simulink model "CASO_EJERCICIO"  (R2019b)
settings: Solver=VariableStepAuto  StartTime=0.0  StopTime=60000  RelTol=1e-3
undefined symbols (not defined in the file): n, p1, p2, p3, Vi
libraries: simulink x12
settings Model: Creator=USUARIO  LastModifiedBy=USUARIO

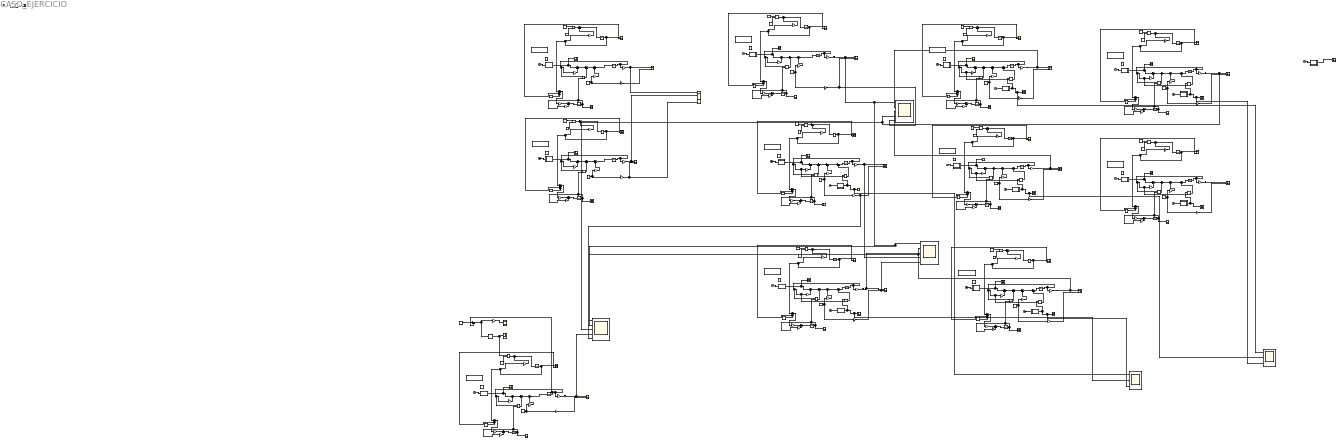
== system CASO_EJERCICIO ==
  COMPARACION MAXIMOS EJERCICIOS PRE Y POST INGESTA : Scope  NumInputPorts=5
  Clock{,1..18,26} (20 alike) : Clock
  Constant{1,3,5,7,9,11,13,15,19,21,29} (11 alike) : Constant  Value=0
  Constant{2,4,6,8,10,12,14,16,20,22,30} (11 alike) : Constant  Value=Vi
  Divide{1..8,10..11,15} (11 alike) : Product  Inputs=*/
  EJERCICIO PREVIO : Scope  NumInputPorts=3
  EJERCICIO TRAS : Scope  NumInputPorts=3
  Error glucémico10 : Scope
  Gain{1,6,8,13,18,20,25,27,32,34,39,41,46,48,53,55,64,68,73,76,105,110} (22 alike) : Gain  Gain=p1
  Gain{3,5,10,12,15,17,22,24,29,31,36,38,43,45,50,52,66,70,72,75,107,109,112} (23 alike) : Gain  Gain=18
  Gain{2,9,21,28,35,42,49,56,65,69,106} (11 alike) : Gain  Gain=p3
  Gain{4,11,16,23,30,37,44,51,67,71,108} (11 alike) : Gain  Gain=n
  Gain{7,14,19,26,33,40,47,54,74,77,111} (11 alike) : Gain  Gain=p2
  Glucosa basal{1..8,10..11,15} (11 alike) : Constant  Value=7
  Grafica ingesta D{1..18,20} (19 alike) : Scope
  Ingesta 75 g1 : MATLAB Function  TreatAsAtomicUnit=on
  Ingesta 75 g10 : MATLAB Function  TreatAsAtomicUnit=on
  Ingesta 75 g11 : MATLAB Function  TreatAsAtomicUnit=on
  Ingesta 75 g15 : MATLAB Function  TreatAsAtomicUnit=on
  Ingesta 75 g2 : MATLAB Function  TreatAsAtomicUnit=on
  Ingesta 75 g3 : MATLAB Function  TreatAsAtomicUnit=on
  Ingesta 75 g4 : MATLAB Function  TreatAsAtomicUnit=on
  Ingesta 75 g5 : MATLAB Function  TreatAsAtomicUnit=on
  Ingesta 75 g6 : MATLAB Function  TreatAsAtomicUnit=on
  Ingesta 75 g7 : MATLAB Function  TreatAsAtomicUnit=on
  Ingesta 75 g8 : MATLAB Function  TreatAsAtomicUnit=on
  Ingesta 75 g9 : MATLAB Function  TreatAsAtomicUnit=on
  Insulina basal{1..8,10..11,15} (11 alike) : Constant  Value=10
  Integrator{1,4,7,10,13,19,22,28,31,43} (10 alike) : Integrator  InitialCondition=10
  Integrator{2,5,8,11,14,17,20,23,29,32,44} (11 alike) : Integrator  InitialCondition=7
  Integrator{3,6,9,12,15..16,18,21,24,30,45} (11 alike) : Integrator
  Integrator33 : Integrator  InitialCondition=-0.000194
  MATLAB Function : MATLAB Function  TreatAsAtomicUnit=on
  MATLAB Function1 : MATLAB Function  TreatAsAtomicUnit=on
  MATLAB Function2 : MATLAB Function  TreatAsAtomicUnit=on
  MATLAB Function3 : MATLAB Function  TreatAsAtomicUnit=on
  MATLAB Function4 : MATLAB Function  TreatAsAtomicUnit=on
  MATLAB Function5 : MATLAB Function  TreatAsAtomicUnit=on
  MATLAB Function6 : MATLAB Function  TreatAsAtomicUnit=on
  MATLAB Function7 : MATLAB Function  TreatAsAtomicUnit=on
  Model Info1 : simulink/Model-Wide Utilities/Model Info  Frame=on  DisplayStringWithTags=|  HorizontalTextAlignment=Center  LeftAlignmentValue=0.5
      | MODELO MODIFICADO
      | 
      | INGESTA SIN INSULINA
      | 
      | PERSONA DIABETICA tipo 1
  Model Info12 : simulink/Model-Wide Utilities/Model Info  Frame=on  DisplayStringWithTags=|  HorizontalTextAlignment=Center  LeftAlignmentValue=0.5
      | MODELO MODIFICADO
      | 
      | INGESTA SIN INSULINA
      | 
      | PERSONA DIABETICA tipo 1
  Model Info13 : simulink/Model-Wide Utilities/Model Info  Frame=on  DisplayStringWithTags=|  HorizontalTextAlignment=Center  LeftAlignmentValue=0.5
      | MODELO MODIFICADO
      | 
      | TRAS INGESTA CON INSULINA
      | 
      | PERSONA DIABETICA
  Model Info14 : simulink/Model-Wide Utilities/Model Info  Frame=on  DisplayStringWithTags=|  HorizontalTextAlignment=Center  LeftAlignmentValue=0.5
      | MODELO MODIFICADO
      | 
      | INGESTA SIN INSULINA
      | 
      | PERSONA DIABETICA tipo 1
  Model Info2 : simulink/Model-Wide Utilities/Model Info  Frame=on  DisplayStringWithTags=|  HorizontalTextAlignment=Center  LeftAlignmentValue=0.5
      | MODELO MODIFICADO
      | 
      | INGESTA SIN INSULINA
      | 
      | PERSONA DIABETICA tipo 1
  Model Info3 : simulink/Model-Wide Utilities/Model Info  Frame=on  DisplayStringWithTags=|  HorizontalTextAlignment=Center  LeftAlignmentValue=0.5
      | MODELO MODIFICADO
      | 
      | INGESTA SIN INSULINA
      | 
      | PERSONA DIABETICA tipo 1
  Model Info4 : simulink/Model-Wide Utilities/Model Info  Frame=on  DisplayStringWithTags=|  HorizontalTextAlignment=Center  LeftAlignmentValue=0.5
      | MODELO MODIFICADO
      | 
      | INGESTA SIN INSULINA
      | 
      | PERSONA DIABETICA tipo 1
  Model Info5 : simulink/Model-Wide Utilities/Model Info  Frame=on  DisplayStringWithTags=|  HorizontalTextAlignment=Center  LeftAlignmentValue=0.5
      | MODELO MODIFICADO
      | 
      | INGESTA SIN INSULINA
      | 
      | PERSONA DIABETICA tipo 1
  Model Info6 : simulink/Model-Wide Utilities/Model Info  Frame=on  DisplayStringWithTags=|  HorizontalTextAlignment=Center  LeftAlignmentValue=0.5
      | MODELO MODIFICADO
      | 
      | INGESTA SIN INSULINA
      | 
      | PERSONA DIABETICA tipo 1
  Model Info7 : simulink/Model-Wide Utilities/Model Info  Frame=on  DisplayStringWithTags=|  HorizontalTextAlignment=Center  LeftAlignmentValue=0.5
      | MODELO MODIFICADO
      | 
      | INGESTA SIN INSULINA
      | 
      | PERSONA DIABETICA tipo 1
  Model Info8 : simulink/Model-Wide Utilities/Model Info  Frame=on  DisplayStringWithTags=|  HorizontalTextAlignment=Center  LeftAlignmentValue=0.5
      | MODELO MODIFICADO
      | 
      | INGESTA SIN INSULINA
      | 
      | PERSONA DIABETICA tipo 1
  PID Controller6 : simulink/Continuous/PID Controller  Controller=PID  Form=Ideal  TimeDomain=Continuous-time  SampleTime=-1  IntegratorMethod=Forward Euler  FilterMethod=Forward Euler  ControllerParametersSource=internal  P=-0.3195  I=0.00033  D=0  UseFilter=on  N=100  TunerSelectOption=Transfer Function Based (PID Tuner App)  InitialConditionSource=internal  InitialConditionForIntegrator=-0.1  InitialConditionForFilter=0  DifferentiatorICPrevScaledInput=0  ExternalReset=none  TrackingMode=off  Kt=1  LimitOutput=off  UpperSaturationLimit=inf  LowerSaturationLimit=-inf  LinearizeAsGain=on  AntiWindupMode=none  Kb=1  POutMin=[]  POutMax=[]  IOutMin=[]  IOutMax=[]  DOutMin=[]  DOutMax=[]  NOutMin=[]  NOutMax=[]  SumOutMin=[]  SumOutMax=[]  SaturationOutMin=[]  SaturationOutMax=[]  PParamMin=[]  PParamMax=[]  IParamMin=[]  IParamMax=[]  DParamMin=[]  DParamMax=[]  NParamMin=[]  NParamMax=[]  KbParamMin=[]  KbParamMax=[]  KtParamMin=[]  KtParamMax=[]  KbOutMin=[]  KbOutMax=[]  KtOutMin=[]  KtOutMax=[]  IntegratorOutMin=[]  IntegratorOutMax=[]  FilterOutMin=[]  FilterOutMax=[]  SumI1OutMin=[]  SumI1OutMax=[]  SumI2OutMin=[]  SumI2OutMax=[]  SumI3OutMin=[]  SumI3OutMax=[]  SumI4OutMin=[]  SumI4OutMax=[]  SumDOutMin=[]  SumDOutMax=[]  DifferentiatorOutMin=[]  DifferentiatorOutMax=[]  FilterDiffOutCoefMin=[]  FilterDiffOutCoefMax=[]  ReciprocalOutMin=[]  ReciprocalOutMax=[]  SumDenOutMin=[]  SumDenOutMax=[]  SumNumOutMin=[]  SumNumOutMax=[]  DivideOutMin=[]  DivideOutMax=[]  IntegratorContinuousStateAttributes=''  IntegratorStateMustResolveToSignalObject=off  IntegratorRTWStateStorageClass=Auto  FilterContinuousStateAttributes=''  FilterStateMustResolveToSignalObject=off  FilterRTWStateStorageClass=Auto  ParallelPVariant=Passthrough  IdealPVariant=InternalParameters  IVariant=InternalParameters  DVariant=InternalParameters  IntegratorVariant=Continuous  SatVariant=Disabled  AWVariant=Passthrough  PCopyVariant=Disabled  TRVariant=Disabled  FdbkBlocksVariant=Forward  IdealPFdbkVariant=Disabled  SatFdbkVariant=Disabled  DerivativeFilterVariant=ContFilter  NVariant=InternalParameters  NCopyVariant=Disabled  FilterICVariant=InternalICsFilter  IntegratorICVariant=InternalICs  ExternalResetVariant=Disabled  TRSumVariant=Passthrough  SumFdbkVariant=Disabled  SumVariant=Sum_PID
  Product{1..17,20} (18 alike) : Product
  Scope : Scope
  Señal de control10 : Scope
  Sum{1..2,4..8,10..19,21..26,28..33,35..40,42..47,49..56,58..60,62..66,92..97} (63 alike) : Sum  Inputs=|+-
  Sum{3,9,20,27,34,41,48,57,61,67,91} (11 alike) : Sum  Inputs=|++
  U (ins. exógena) cte{1..8,10} (9 alike) : Constant  Value=0
  U (ins. exógena) cte11 : Constant  Value=0.185
  glucosa tras ingesta1 : Scope  NumInputPorts=5
  glucosa tras ingesta{2..10,12,19} (11 alike) : Scope  NumInputPorts=2
  glucosa tras ingesta11 : Scope  NumInputPorts=5
  glucosa tras ingesta14 : Scope  NumInputPorts=4
  grafica insulina{1..8,12,14..15} (11 alike) : Scope  NumInputPorts=2
  insulina activa{1..8,10..11,15} (11 alike) : Scope
  referencia glucosa = Gb6 : Constant  Value=7
  wires:
  Integrator29/1 -> Gain66/1, Product10/1, Gain64/1  "G(t)"
  Divide10/1 -> Sum66/1
  Gain73/1 -> Sum61/2
  Gain74/1 -> Sum62/2
  Constant22/1 -> Divide11/2
  Sum60/1 -> Sum63/1
  Glucosa basal11/1 -> Gain73/1, Gain72/1  "glucosa basal"
  Integrator33/1 -> insulina activa11/1, Product11/2, Gain74/1  "X(t)"
  Sum55/1 -> Gain65/1
  U (ins. exógena) cte11/1 -> Divide11/1
  Gain77/1 -> Sum58/2
  Gain64/1 -> Sum56/2
  Sum66/1 -> Integrator28/1
  Gain66/1 -> glucosa tras ingesta9/1, glucosa tras ingesta14/1  "INGESTA PACIENTE DIABETICO"
  Sum63/1 -> Sum61/1
  Clock10/1 -> Ingesta 75 g10/1(in)
  Gain72/1 -> glucosa tras ingesta14/4, glucosa tras ingesta10/2  "glucosa basal"
  Integrator31/1 -> grafica insulina12/1, Gain71/1, Sum59/1  "I(t)"
  Gain71/1 -> Sum64/2
  Insulina basal11/1 -> grafica insulina12/2, Sum59/2  "insulina basal"
  Gain67/1 -> Sum66/2
  Product11/1 -> Sum63/2
  Sum65/1 -> Sum57/1
  Gain68/1 -> Sum60/2
  U (ins. exógena) cte10/1 -> Divide10/1
  Integrator28/1 -> grafica insulina14/1, Gain67/1, Sum55/1  "I(t)"
  Ingesta 75 g10/1(D) -> Grafica ingesta D10/1, Sum56/1
  Ingesta 75 g11/1(D) -> Grafica ingesta D11/1, Sum60/1
  Sum58/1 -> Integrator30/1
  Sum57/1 -> Integrator29/1
  Integrator30/1 -> insulina activa10/1, Product10/2, Gain77/1  "X(t)"
  Glucosa basal10/1 -> Gain76/1, Gain75/1  "glucosa basal"
  Gain75/1 -> glucosa tras ingesta9/2  "glucosa basal diabetico"
  Sum59/1 -> Gain69/1
  Integrator32/1 -> Gain70/1, Product11/1, Gain68/1  "G(t)"
  Sum56/1 -> Sum65/1
  Sum62/1 -> Integrator33/1
  Product10/1 -> Sum65/2
  Gain65/1 -> Sum58/1
  Divide11/1 -> Sum64/1
  Constant20/1 -> Divide10/2
  Sum61/1 -> Integrator32/1
  Gain69/1 -> Sum62/1
  Gain70/1 -> glucosa tras ingesta14/2, glucosa tras ingesta10/1  "Ingesta con insulina"
  Sum64/1 -> Integrator31/1
  Insulina basal10/1 -> grafica insulina14/2, Sum55/2  "insulina basal"
  Clock11/1 -> Ingesta 75 g11/1(in)
  Gain76/1 -> Sum57/2
  Gain5/1 -> glucosa tras ingesta1/5, glucosa tras ingesta2/2  "glucosa basal diabetico"
  Glucosa basal1/1 -> Gain6/1, Gain5/1  "glucosa basal"
  Sum4/1 -> Integrator3/1
  Gain6/1 -> Sum3/2
  Integrator2/1 -> Gain3/1, Product1/1, Gain1/1  "G(t)"
  Divide1/1 -> Sum6/1
  Integrator1/1 -> grafica insulina1/1, Gain4/1, Sum1/1  "I(t)"
  Integrator3/1 -> insulina activa1/1, Product1/2, Gain7/1  "X(t)"
  Sum5/1 -> Sum3/1
  Ingesta 75 g1/1(D) -> Grafica ingesta D1/1, Sum2/1
  U (ins. exógena) cte1/1 -> Divide1/1
  Gain4/1 -> Sum6/2
  Constant2/1 -> Divide1/2
  Gain2/1 -> Sum4/1
  Product1/1 -> Sum5/2
  Gain3/1 -> glucosa tras ingesta11/1, COMPARACION MAXIMOS EJERCICIOS PRE Y POST INGESTA/1, glucosa tras ingesta1/1, glucosa tras ingesta2/1  "Ingesta"
  Clock1/1 -> Ingesta 75 g1/1(in)
  Gain1/1 -> Sum2/2
  Gain7/1 -> Sum4/2
  Sum6/1 -> Integrator1/1
  Sum1/1 -> Gain2/1
  Insulina basal1/1 -> grafica insulina1/2, Sum1/2  "insulina basal"
  Sum2/1 -> Sum5/1
  Sum3/1 -> Integrator2/1
  Sum10/1 -> Integrator6/1
  U (ins. exógena) cte2/1 -> Divide2/1
  Gain10/1 -> glucosa tras ingesta11/4, glucosa tras ingesta3/1  "Ejercicio previo a la ingesta: Periodo corto"
  Product2/1 -> Sum11/2
  Sum11/1 -> Sum9/1
  Gain12/1 -> COMPARACION MAXIMOS EJERCICIOS PRE Y POST INGESTA/5, glucosa tras ingesta3/2  "glucosa basal diabetico"
  Integrator5/1 -> Gain10/1, Product2/1, Product3/2, Gain8/1  "G(t)"
  Integrator4/1 -> grafica insulina2/1, Gain11/1, Sum7/1  "I(t)"
  Glucosa basal2/1 -> Gain13/1, Gain12/1  "glucosa basal"
  Integrator6/1 -> insulina activa2/1, Product2/2, Gain14/1  "X(t)"
  Divide2/1 -> Sum12/1
  Insulina basal2/1 -> grafica insulina2/2, Sum7/2  "insulina basal"
  Gain13/1 -> Sum9/2
  Sum8/1 -> Sum11/1
  Gain9/1 -> Sum10/1
  Gain8/1 -> Sum8/2
  Gain11/1 -> Sum12/2
  Sum7/1 -> Gain9/1
  Ingesta 75 g2/1(D) -> Grafica ingesta D2/1, Sum8/1
  Sum12/1 -> Integrator4/1
  Clock2/1 -> Ingesta 75 g2/1(in)
  Gain14/1 -> Sum10/2
  Constant4/1 -> Divide2/2
  Sum9/1 -> Sum13/1
  Sum13/1 -> Integrator5/1
  Product3/1 -> Sum13/2
  Clock/1 -> MATLAB Function/1(in)
  MATLAB Function/1(Ej) -> Product3/1, EJERCICIO PREVIO/1, Grafica ingesta D3/1  "Ejercicio previo a la ingesta: Periodo corto"
  MATLAB Function1/1(Ej) -> Product5/1, EJERCICIO TRAS/1, Grafica ingesta D5/1  "Ejercicio tras ingesta: Periodo corto"
  Gain17/1 -> glucosa tras ingesta4/2  "glucosa basal diabetico"
  Integrator8/1 -> Gain15/1, Product4/1, Product5/2, Gain20/1  "G(t)"
  Sum15/1 -> Sum20/1
  Product4/1 -> Sum15/2
  Glucosa basal3/1 -> Gain18/1, Gain17/1  "glucosa basal"
  Integrator7/1 -> grafica insulina3/1, Gain16/1, Sum18/1  "I(t)"
  Gain18/1 -> Sum20/2
  Insulina basal3/1 -> grafica insulina3/2, Sum18/2  "insulina basal"
  Constant6/1 -> Divide3/2
  Sum16/1 -> Integrator7/1
  Clock4/1 -> Ingesta 75 g3/1(in)
  Sum18/1 -> Gain21/1
  Ingesta 75 g3/1(D) -> Grafica ingesta D4/1, Sum19/1
  Gain16/1 -> Sum16/2
  Gain20/1 -> Sum19/2
  Gain21/1 -> Sum14/1
  Sum19/1 -> Sum15/1
  Sum20/1 -> Sum17/1
  Gain15/1 -> glucosa tras ingesta1/2, glucosa tras ingesta4/1  "Ejercicio tras ingesta: Periodo corto"
  U (ins. exógena) cte3/1 -> Divide3/1
  Gain19/1 -> Sum14/2
  Sum14/1 -> Integrator9/1
  Sum17/1 -> Integrator8/1
  Clock3/1 -> MATLAB Function1/1(in)
  Integrator9/1 -> insulina activa3/1, Product4/2, Gain19/1  "X(t)"
  Product5/1 -> Sum17/2
  Divide3/1 -> Sum16/1
  MATLAB Function2/1(Ej) -> Product7/1, EJERCICIO TRAS/2, Grafica ingesta D7/1  "Ejercicio tras ingesta: Periodo largo"
  Gain24/1 -> glucosa tras ingesta5/2  "glucosa basal diabetico"
  Integrator11/1 -> Gain22/1, Product6/1, Product7/2, Gain27/1  "G(t)"
  Sum22/1 -> Sum27/1
  Product6/1 -> Sum22/2
  Glucosa basal4/1 -> Gain25/1, Gain24/1  "glucosa basal"
  Integrator10/1 -> grafica insulina4/1, Gain23/1, Sum25/1  "I(t)"
  Gain25/1 -> Sum27/2
  Insulina basal4/1 -> grafica insulina4/2, Sum25/2  "insulina basal"
  Constant8/1 -> Divide4/2
  Sum23/1 -> Integrator10/1
  Clock6/1 -> Ingesta 75 g4/1(in)
  Sum25/1 -> Gain28/1
  Ingesta 75 g4/1(D) -> Grafica ingesta D6/1, Sum26/1
  Gain23/1 -> Sum23/2
  Gain27/1 -> Sum26/2
  Gain28/1 -> Sum21/1
  Sum26/1 -> Sum22/1
  Sum27/1 -> Sum24/1
  Gain22/1 -> glucosa tras ingesta1/3, glucosa tras ingesta5/1  "Ejercicio tras ingesta: Periodo largo"
  U (ins. exógena) cte4/1 -> Divide4/1
  Gain26/1 -> Sum21/2
  Sum21/1 -> Integrator12/1
  Sum24/1 -> Integrator11/1
  Clock5/1 -> MATLAB Function2/1(in)
  Integrator12/1 -> insulina activa4/1, Product6/2, Gain26/1  "X(t)"
  Product7/1 -> Sum24/2
  Divide4/1 -> Sum23/1
  MATLAB Function3/1(Ej) -> Product9/1, EJERCICIO TRAS/3, Grafica ingesta D9/1  "Ejercicio tras ingesta: Periodo muy largo"
  Gain31/1 -> glucosa tras ingesta6/2  "glucosa basal diabetico"
  Integrator14/1 -> Gain29/1, Product8/1, Product9/2, Gain34/1  "G(t)"
  Sum29/1 -> Sum34/1
  Product8/1 -> Sum29/2
  Glucosa basal5/1 -> Gain32/1, Gain31/1  "glucosa basal"
  Integrator13/1 -> grafica insulina5/1, Gain30/1, Sum32/1  "I(t)"
  Gain32/1 -> Sum34/2
  Insulina basal5/1 -> grafica insulina5/2, Sum32/2  "insulina basal"
  Constant10/1 -> Divide5/2
  Sum30/1 -> Integrator13/1
  Clock8/1 -> Ingesta 75 g5/1(in)
  Sum32/1 -> Gain35/1
  Ingesta 75 g5/1(D) -> Grafica ingesta D8/1, Sum33/1
  Gain30/1 -> Sum30/2
  Gain34/1 -> Sum33/2
  Gain35/1 -> Sum28/1
  Sum33/1 -> Sum29/1
  Sum34/1 -> Sum31/1
  Gain29/1 -> glucosa tras ingesta1/4, COMPARACION MAXIMOS EJERCICIOS PRE Y POST INGESTA/3, glucosa tras ingesta6/1  "Ejercicio tras ingesta: Periodo muy largo"
  U (ins. exógena) cte5/1 -> Divide5/1
  Gain33/1 -> Sum28/2
  Sum28/1 -> Integrator15/1
  Sum31/1 -> Integrator14/1
  Clock7/1 -> MATLAB Function3/1(in)
  Integrator15/1 -> insulina activa5/1, Product8/2, Gain33/1  "X(t)"
  Product9/1 -> Sum31/2
  Divide5/1 -> Sum30/1
  MATLAB Function4/1(Ej) -> Product13/1, Grafica ingesta D13/1
  Gain38/1 -> glucosa tras ingesta7/2  "glucosa basal diabetico"
  Integrator17/1 -> Gain36/1, Product12/1, Product13/2, Gain41/1  "G(t)"
  Sum36/1 -> Sum41/1
  Product12/1 -> Sum36/2
  Glucosa basal6/1 -> Gain39/1, Gain38/1  "glucosa basal"
  Integrator16/1 -> grafica insulina6/1, Gain37/1, Sum39/1  "I(t)"
  Gain39/1 -> Sum41/2
  Insulina basal6/1 -> grafica insulina6/2, Sum39/2  "insulina basal"
  Constant12/1 -> Divide6/2
  Sum37/1 -> Integrator16/1
  Clock12/1 -> Ingesta 75 g6/1(in)
  Sum39/1 -> Gain42/1
  Ingesta 75 g6/1(D) -> Grafica ingesta D12/1, Sum40/1
  Gain37/1 -> Sum37/2
  Gain41/1 -> Sum40/2
  Gain42/1 -> Sum35/1
  Sum40/1 -> Sum36/1
  Sum41/1 -> Sum38/1
  Gain36/1 -> glucosa tras ingesta7/1  "Ejercicio tras ingesta: Periodo 4"
  U (ins. exógena) cte6/1 -> Divide6/1
  Gain40/1 -> Sum35/2
  Sum35/1 -> Integrator18/1
  Sum38/1 -> Integrator17/1
  Clock9/1 -> MATLAB Function4/1(in)
  Integrator18/1 -> insulina activa6/1, Product12/2, Gain40/1  "X(t)"
  Product13/1 -> Sum38/2
  Divide6/1 -> Sum37/1
  MATLAB Function5/1(Ej) -> Product15/1, EJERCICIO PREVIO/2, Grafica ingesta D15/1  "Ejercicio previo a la ingesta: Periodo largo"
  Gain45/1 -> glucosa tras ingesta11/5, glucosa tras ingesta8/2  "glucosa basal diabetico"
  Integrator20/1 -> Gain43/1, Product14/1, Product15/2, Gain48/1  "G(t)"
  Sum43/1 -> Sum48/1
  Product14/1 -> Sum43/2
  Glucosa basal7/1 -> Gain46/1, Gain45/1  "glucosa basal"
  Integrator19/1 -> grafica insulina7/1, Gain44/1, Sum46/1  "I(t)"
  Gain46/1 -> Sum48/2
  Insulina basal7/1 -> grafica insulina7/2, Sum46/2  "insulina basal"
  Constant14/1 -> Divide7/2
  Sum44/1 -> Integrator19/1
  Clock14/1 -> Ingesta 75 g7/1(in)
  Sum46/1 -> Gain49/1
  Ingesta 75 g7/1(D) -> Grafica ingesta D14/1, Sum47/1
  Gain44/1 -> Sum44/2
  Gain48/1 -> Sum47/2
  Gain49/1 -> Sum42/1
  Sum47/1 -> Sum43/1
  Sum48/1 -> Sum45/1
  Gain43/1 -> glucosa tras ingesta11/3, glucosa tras ingesta8/1  "Ejercicio previo a la ingesta: Periodo largo"
  U (ins. exógena) cte7/1 -> Divide7/1
  Gain47/1 -> Sum42/2
  Sum42/1 -> Integrator21/1
  Sum45/1 -> Integrator20/1
  Clock13/1 -> MATLAB Function5/1(in)
  Integrator21/1 -> insulina activa7/1, Product14/2, Gain47/1  "X(t)"
  Product15/1 -> Sum45/2
  Divide7/1 -> Sum44/1
  Gain53/1 -> Sum67/2
  Product16/1 -> Sum50/2
  Integrator22/1 -> grafica insulina8/1, Gain51/1, Sum53/1  "I(t)"
  Glucosa basal8/1 -> Gain53/1, Gain52/1  "glucosa basal"
  Divide8/1 -> Sum51/1
  Gain52/1 -> glucosa tras ingesta12/2  "glucosa basal diabetico"
  MATLAB Function6/1(Ej) -> Product17/1, EJERCICIO PREVIO/3, Grafica ingesta D17/1  "Ejercicio previo a la ingesta: Periodo muy largo"
  Product17/1 -> Sum52/2
  Insulina basal8/1 -> grafica insulina8/2, Sum53/2  "insulina basal"
  Gain55/1 -> Sum54/2
  Gain56/1 -> Sum49/1
  Ingesta 75 g8/1(D) -> Grafica ingesta D16/1, Sum54/1
  Sum53/1 -> Gain56/1
  Sum51/1 -> Integrator22/1
  Constant16/1 -> Divide8/2
  Sum67/1 -> Sum52/1
  Gain50/1 -> glucosa tras ingesta11/2, COMPARACION MAXIMOS EJERCICIOS PRE Y POST INGESTA/2, glucosa tras ingesta12/1  "Ejercicio previo a la ingesta: Periodo muy largo"
  Sum52/1 -> Integrator23/1
  Sum49/1 -> Integrator24/1
  Gain54/1 -> Sum49/2
  Integrator24/1 -> insulina activa8/1, Product16/2, Gain54/1  "X(t)"
  U (ins. exógena) cte8/1 -> Divide8/1
  Clock16/1 -> Ingesta 75 g8/1(in)
  Sum50/1 -> Sum67/1
  Integrator23/1 -> Gain50/1, Product16/1, Product17/2, Gain55/1  "G(t)"
  Sum54/1 -> Sum50/1
  Clock15/1 -> MATLAB Function6/1(in)
  Gain51/1 -> Sum51/2
  Clock17/1 -> Ingesta 75 g9/1(in)
  Ingesta 75 g9/1(D) -> Grafica ingesta D18/1
  Sum95/1 -> PID Controller6/1, Gain112/1  "error(ref-actual)"
  Gain112/1 -> Error glucémico10/1  "Error regulador P"
  Sum97/1 -> Sum93/1
  Gain105/1 -> Sum97/2
  Integrator43/1 -> grafica insulina15/1, Gain108/1, Sum96/1  "I(t)"
  Glucosa basal15/1 -> Gain110/1, Gain109/1  "glucosa basal"
  Integrator44/1 -> Sum95/2, Gain107/1, Product20/1, Gain105/1  "G(t)"
  Product20/1 -> Sum93/2
  PID Controller6/1 -> Divide15/1, Señal de control10/1  "Control regulador P"
  Gain106/1 -> Sum92/1
  Sum96/1 -> Gain106/1
  Ingesta 75 g15/1(D) -> Grafica ingesta D20/1, Sum97/1
  Sum91/1 -> Integrator44/1
  Sum92/1 -> Integrator45/1
  Gain110/1 -> Sum91/2
  Sum93/1 -> Sum91/1
  Gain107/1 -> COMPARACION MAXIMOS EJERCICIOS PRE Y POST INGESTA/4, glucosa tras ingesta19/1  "Con regulador"
  Divide15/1 -> Sum94/1
  Sum94/1 -> Integrator43/1
  Gain109/1 -> glucosa tras ingesta19/2  "glucosa basal diabetico"
  referencia glucosa = Gb6/1 -> Sum95/1  "referencia"
  Gain111/1 -> Sum92/2
  Gain108/1 -> Sum94/2
  Clock26/1 -> Ingesta 75 g15/1(in)
  Constant30/1 -> Divide15/2
  Integrator45/1 -> insulina activa15/1, Product20/2, Gain111/1  "X(t)"
  Insulina basal15/1 -> grafica insulina15/2, Sum96/2  "insulina basal"
  Clock18/1 -> MATLAB Function7/1(in)
  MATLAB Function7/1(Ej) -> Scope/1

== matlab function CASO_EJERCICIO/Ingesta 75 g1 ==
  data: in input; D output
function D = comida(in)
% Variables de entrada en la funcion
t = in(1) %- 8*60*60; % Ajuste para iniciar a las 8 de la mañana
 
% Parámetros del modelo
Ag = 0.8; % adimensional
Tmaxi = 55*60; % s
Vg = 13.79; % L
Tmaxg = 40*60; % s
t1 = 0;
Dg = 0;
f = 1000/180; % factor de conversión de g a mmol
 
% Comidas (perturbaciones) a lo largo de un día
if t >= 180*60 && t < 480*60 % ingesta de 75 g de HC
    t1 = 180*60;
    Dg = 50*f;
end
 
% Ecuación
D = (Dg*Ag*(t-t1)*exp(-(t-t1)/Tmaxi))/(Vg*Tmaxg^2);

== matlab function CASO_EJERCICIO/Ingesta 75 g2 ==
  data: in input; D output
function D = comida(in)
% Variables de entrada en la funcion
t = in(1) %- 8*60*60; % Ajuste para iniciar a las 8 de la mañana
 
% Parámetros del modelo
Ag = 0.8; % adimensional
Tmaxi = 55*60; % s
Vg = 13.79; % L
Tmaxg = 40*60; % s
t1 = 0;
Dg = 0;
f = 1000/180; % factor de conversión de g a mmol
 
% Comidas (perturbaciones) a lo largo de un día
if t >= 180*60 && t < 480*60 % ingesta de 75 g de HC
    t1 = 180*60;
    Dg = 50*f;
end
 
% Ecuación
D = (Dg*Ag*(t-t1)*exp(-(t-t1)/Tmaxi))/(Vg*Tmaxg^2);

== matlab function CASO_EJERCICIO/MATLAB Function ==
  data: in input; Ej output
function Ej  = ejercicio(in)
% Variables de entrada en la funcion
t = in(1);
%Parametros del modelo
cons = 0.005/60;
%Ejercicio (perturbaciones) a lo largo de un día

if t>=0 && t<120*60 %ejercicio 1 h
 Ej=0;
elseif t>=120*60 && t<180*60 %ejercicio 1 h
 Ej=cons+ 0.005/60;
else
 Ej=cons/4;
end

== matlab function CASO_EJERCICIO/Ingesta 75 g3 ==
  data: in input; D output
function D = comida(in)
% Variables de entrada en la funcion
t = in(1) %- 8*60*60; % Ajuste para iniciar a las 8 de la mañana
 
% Parámetros del modelo
Ag = 0.8; % adimensional
Tmaxi = 55*60; % s
Vg = 13.79; % L
Tmaxg = 40*60; % s
t1 = 0;
Dg = 0;
f = 1000/180; % factor de conversión de g a mmol
 
% Comidas (perturbaciones) a lo largo de un día
if t >= 180*60 && t < 480*60 % ingesta de 75 g de HC
    t1 = 180*60;
    Dg = 50*f;
end
 
% Ecuación
D = (Dg*Ag*(t-t1)*exp(-(t-t1)/Tmaxi))/(Vg*Tmaxg^2);

== matlab function CASO_EJERCICIO/MATLAB Function1 ==
  data: in input; Ej output
function Ej  = ejercicio(in)
% Variables de entrada en la funcion
t = in(1);
%Parametros del modelo
cons = 0.005/60;
%Ejercicio (perturbaciones) a lo largo de un día

if t>=0 && t<240*60 %ejercicio 1 h
 Ej=0;
elseif t>=240*60 && t<300*60 %ejercicio 1 h
 Ej=cons+ 0.005/60;
else
 Ej=cons/4;
end

== matlab function CASO_EJERCICIO/Ingesta 75 g4 ==
  data: in input; D output
function D = comida(in)
% Variables de entrada en la funcion
t = in(1) %- 8*60*60; % Ajuste para iniciar a las 8 de la mañana
 
% Parámetros del modelo
Ag = 0.8; % adimensional
Tmaxi = 55*60; % s
Vg = 13.79; % L
Tmaxg = 40*60; % s
t1 = 0;
Dg = 0;
f = 1000/180; % factor de conversión de g a mmol
 
% Comidas (perturbaciones) a lo largo de un día
if t >= 180*60 && t < 480*60 % ingesta de 75 g de HC
    t1 = 180*60;
    Dg = 50*f;
end
 
% Ecuación
D = (Dg*Ag*(t-t1)*exp(-(t-t1)/Tmaxi))/(Vg*Tmaxg^2);

== matlab function CASO_EJERCICIO/MATLAB Function2 ==
  data: in input; Ej output
function Ej  = ejercicio(in)
% Variables de entrada en la funcion
t = in(1);
%Parametros del modelo
cons = 0.005/60;
%Ejercicio (perturbaciones) a lo largo de un día

if t>=0 && t<240*60 %ejercicio 1 h
 Ej=0;
elseif t>=240*60 && t<360*60 %ejercicio 1 h
 Ej=cons+ 0.005/60;
else
 Ej=cons/2;
end

== matlab function CASO_EJERCICIO/Ingesta 75 g5 ==
  data: in input; D output
function D = comida(in)
% Variables de entrada en la funcion
t = in(1) %- 8*60*60; % Ajuste para iniciar a las 8 de la mañana
 
% Parámetros del modelo
Ag = 0.8; % adimensional
Tmaxi = 55*60; % s
Vg = 13.79; % L
Tmaxg = 40*60; % s
t1 = 0;
Dg = 0;
f = 1000/180; % factor de conversión de g a mmol
 
% Comidas (perturbaciones) a lo largo de un día
if t >= 180*60 && t < 480*60 % ingesta de 75 g de HC
    t1 = 180*60;
    Dg = 50*f;
end
 
% Ecuación
D = (Dg*Ag*(t-t1)*exp(-(t-t1)/Tmaxi))/(Vg*Tmaxg^2);

== matlab function CASO_EJERCICIO/MATLAB Function3 ==
  data: in input; Ej output
function Ej  = ejercicio(in)
% Variables de entrada en la funcion
t = in(1);
%Parametros del modelo
cons = 0.005/60;
%Ejercicio (perturbaciones) a lo largo de un día

if t>=0 && t<240*60 %ejercicio 1 h
 Ej=0;
elseif t>=240*60 && t<480*60 %ejercicio 1 h
 Ej=cons+ 0.005/60;
else
 Ej=cons;
end

== matlab function CASO_EJERCICIO/Ingesta 75 g10 ==
  data: in input; D output
function D = comida(in)
% Variables de entrada en la funcion
t = in(1) %- 8*60*60; % Ajuste para iniciar a las 8 de la mañana
 
% Parámetros del modelo
Ag = 0.8; % adimensional
Tmaxi = 55*60; % s
Vg = 13.79; % L
Tmaxg = 40*60; % s
t1 = 0;
Dg = 0;
f = 1000/180; % factor de conversión de g a mmol
 
% Comidas (perturbaciones) a lo largo de un día
if t >= 180*60 && t < 480*60 % ingesta de 75 g de HC
    t1 = 180*60;
    Dg = 50*f;
end
 
% Ecuación
D = (Dg*Ag*(t-t1)*exp(-(t-t1)/Tmaxi))/(Vg*Tmaxg^2);

== matlab function CASO_EJERCICIO/Ingesta 75 g11 ==
  data: in input; D output
function D = comida(in)
% Variables de entrada en la funcion
t = in(1) %- 8*60*60; % Ajuste para iniciar a las 8 de la mañana
 
% Parámetros del modelo
Ag = 0.8; % adimensional
Tmaxi = 55*60; % s
Vg = 13.79; % L
Tmaxg = 40*60; % s
t1 = 0;
Dg = 0;
f = 1000/180; % factor de conversión de g a mmol
 
% Comidas (perturbaciones) a lo largo de un día
if t >= 180*60 && t < 480*60 % ingesta de 75 g de HC
    t1 = 180*60;
    Dg = 50*f;
end
 
% Ecuación
D = (Dg*Ag*(t-t1)*exp(-(t-t1)/Tmaxi))/(Vg*Tmaxg^2);

== matlab function CASO_EJERCICIO/Ingesta 75 g6 ==
  data: in input; D output
function D = comida(in)
% Variables de entrada en la funcion
t = in(1) %- 8*60*60; % Ajuste para iniciar a las 8 de la mañana
 
% Parámetros del modelo
Ag = 0.8; % adimensional
Tmaxi = 55*60; % s
Vg = 13.79; % L
Tmaxg = 40*60; % s
t1 = 0;
Dg = 0;
f = 1000/180; % factor de conversión de g a mmol
 
% Comidas (perturbaciones) a lo largo de un día
if t >= 180*60 && t < 480*60 % ingesta de 75 g de HC
    t1 = 180*60;
    Dg = 50*f;
end
 
% Ecuación
D = (Dg*Ag*(t-t1)*exp(-(t-t1)/Tmaxi))/(Vg*Tmaxg^2);

== matlab function CASO_EJERCICIO/MATLAB Function4 ==
  data: in input; Ej output
function Ej  = ejercicio(in)
% Variables de entrada en la funcion
t = in(1);
%Parametros del modelo
cons = 0.005/60;
%Ejercicio (perturbaciones) a lo largo de un día

if t>=0 && t<240*60 %ejercicio 1 h
 Ej=0;
elseif t>=240*60 && t<480*60 %ejercicio 1 h
 Ej=cons+ 0.005/60;
else
 Ej=cons;
end

== matlab function CASO_EJERCICIO/Ingesta 75 g7 ==
  data: in input; D output
function D = comida(in)
% Variables de entrada en la funcion
t = in(1) %- 8*60*60; % Ajuste para iniciar a las 8 de la mañana
 
% Parámetros del modelo
Ag = 0.8; % adimensional
Tmaxi = 55*60; % s
Vg = 13.79; % L
Tmaxg = 40*60; % s
t1 = 0;
Dg = 0;
f = 1000/180; % factor de conversión de g a mmol
 
% Comidas (perturbaciones) a lo largo de un día
if t >= 180*60 && t < 480*60 % ingesta de 75 g de HC
    t1 = 180*60;
    Dg = 50*f;
end
 
% Ecuación
D = (Dg*Ag*(t-t1)*exp(-(t-t1)/Tmaxi))/(Vg*Tmaxg^2);

== matlab function CASO_EJERCICIO/MATLAB Function5 ==
  data: in input; Ej output
function Ej  = ejercicio(in)
% Variables de entrada en la funcion
t = in(1);
%Parametros del modelo
cons = 0.005/60;
%Ejercicio (perturbaciones) a lo largo de un día

if t>=0 && t<60*60 %ejercicio 1 h
 Ej=0;
elseif t>=60*60 && t<180*60 %ejercicio 2 h
 Ej=cons+ 0.005/60;
else
 Ej=cons/2;
end

== matlab function CASO_EJERCICIO/Ingesta 75 g8 ==
  data: in input; D output
function D = comida(in)
% Variables de entrada en la funcion
t = in(1) %- 8*60*60; % Ajuste para iniciar a las 8 de la mañana
 
% Parámetros del modelo
Ag = 0.8; % adimensional
Tmaxi = 55*60; % s
Vg = 13.79; % L
Tmaxg = 40*60; % s
t1 = 0;
Dg = 0;
f = 1000/180; % factor de conversión de g a mmol
 
% Comidas (perturbaciones) a lo largo de un día
if t >= 180*60 && t < 480*60 % ingesta de 75 g de HC
    t1 = 180*60;
    Dg = 50*f;
end
 
% Ecuación
D = (Dg*Ag*(t-t1)*exp(-(t-t1)/Tmaxi))/(Vg*Tmaxg^2);

== matlab function CASO_EJERCICIO/MATLAB Function6 ==
  data: in input; Ej output
function Ej  = ejercicio(in)
% Variables de entrada en la funcion
t = in(1);
%Parametros del modelo
cons = 0.005/60;
%Ejercicio (perturbaciones) a lo largo de un día

if t>=0 && t<0.1*60 %ejercicio 1 h
 Ej=0;
elseif t>=0.1*60 && t<180*60 %ejercicio 1 h
 Ej=cons+ 0.005/60;
else
 Ej=cons;
end

== matlab function CASO_EJERCICIO/Ingesta 75 g9 ==
  data: in input; D output
function D = comida(in)
% Variables de entrada en la funcion
t = in(1) %- 8*60*60; % Ajuste para iniciar a las 8 de la mañana
 
% Parámetros del modelo
Ag = 0.8; % adimensional
Tmaxi = 55*60; % s
Vg = 13.79; % L
Tmaxg = 40*60; % s
t1 = 0;
Dg = 0;
f = 1000/180; % factor de conversión de g a mmol
 
% Comidas (perturbaciones) a lo largo de un día
if t >= 180*60 && t < 580*60 % ingesta de 75 g de HC
    t1 = 180*60;
    Dg = 50*f;
end
 
% Ecuación
D = (Dg*Ag*(t-t1)*exp(-(t-t1)/Tmaxi))/(Vg*Tmaxg^2);

== matlab function CASO_EJERCICIO/MATLAB Function7 ==
  data: in input; Ej output
function Ej  = ejercicio(in)
% Variables de entrada en la funcion
t = in(1);
%Parametros del modelo
cons = 0.005/60;
%Ejercicio (perturbaciones) a lo largo de un día

if t>=180*60 && t<240*60 %ejercicio 1 h
 Ej=cons+ 0.005/60;
else
  Ej =0;
end

== matlab function CASO_EJERCICIO/Ingesta 75 g15 ==
  data: in input; D output
function D = comida(in)
% Variables de entrada en la funcion
t = in(1) %- 8*60*60; % Ajuste para iniciar a las 8 de la mañana
 
% Parámetros del modelo
Ag = 0.8; % adimensional
Tmaxi = 55*60; % s
Vg = 13.79; % L
Tmaxg = 40*60; % s
t1 = 0;
Dg = 0;
f = 1000/180; % factor de conversión de g a mmol
 
% Comidas (perturbaciones) a lo largo de un día
if t >= 180*60 && t < 480*60 % ingesta de 75 g de HC
    t1 = 180*60;
    Dg = 50*f;
end
 
% Ecuación
D = (Dg*Ag*(t-t1)*exp(-(t-t1)/Tmaxi))/(Vg*Tmaxg^2);
